simulink model "snell_th"  (R2018b)
settings: Solver=ode8  StartTime=0.0  StopTime=0  RelTol=1e-3
libraries: find6DOFSnell_cl x1
settings Model: Creator=asiddiq2  LastModifiedBy=asiddiq2

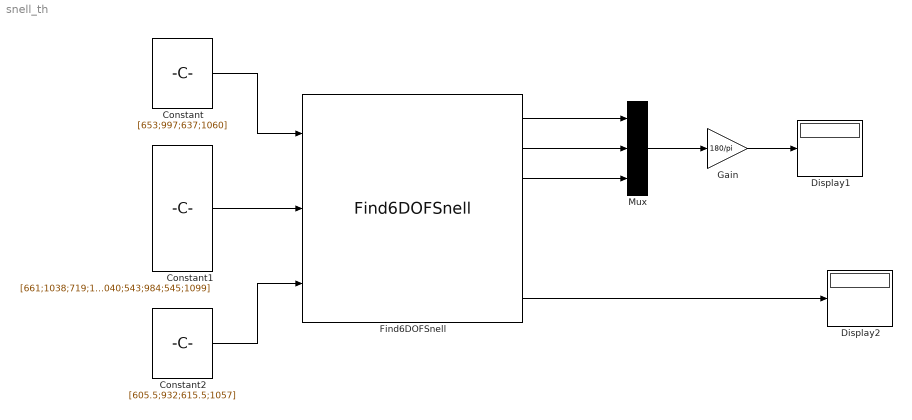
== system snell_th ==
  Constant : Constant  Value=[653;997;637;1060]  VectorParams1D=off
  Constant1 : Constant  Value=[661;1038;719;1040;543;984;545;1099]  VectorParams1D=off
  Constant2 : Constant  Value=[605.5;932;615.5;1057]  VectorParams1D=off
  Display1 : Display
  Display2 : Display
  Find6DOFSnell : find6DOFSnell_cl/Find6DOFSnell  imageDims_px=params.sideImageSize_px.Value  initialCoMPositionVec_cm=params.initCoMPosVec_cm.Value  indxOfRefVec=params.indexOfRefractionAGW.Value  glassThickness_cm=params.glassThickness_cm.Value  prscGlassThick_cm=(3/16)*2.54  cameraFOVAngles_deg=params.cameraFOV_deg.Value  sideEulerAngles_deg=params.sideCamEulAng_deg.Value  sideCamPositionVec_cm=params.sideCamPosVec_cm.Value  sideCamDistToGlass_cm=params.sideDistancetoGlass_cm.Value  botEulerAngles_deg=params.botCamEulAng_deg.Value  botCamPositionVec_cm=params.botCamPosVec_cm.Value  botCamDistToGlass_cm=params.botDistancetoGlass_cm.Value  slantEulerAngles_deg=params.prscpeCamEulAng_deg.Value  slantCamPositionVec_cm=params.prscpeCamPosVec_cm.Value  slantCamDistToGlass_cm=params.prscpeDistancetoGlass_cm.Value  sideSeparation_cm=params.sideDotSepDist_cm.Value  sidePositionVecBF_cm=params.sideDotPosVec_cm.Value  bottomASeparation_cm=params.botADotSepDist_cm.Value  botAPositionVecBF_cm=params.botADotPosVec_cm.Value  bottomBSeparation_cm=params.botBDotSepDist_cm.Value  botBPositionVecBF_cm=params.botBDotPosVec_cm.Value  topSeparation_cm=params.topDotSepDist_cm.Value  topPositionVecBF_cm=params.topDotPosVec_cm.Value
  Gain : Gain  Gain=180/pi
  Mux : Mux  Inputs=3
  wires:
  Constant/1 -> Find6DOFSnell/1
  Constant1/1 -> Find6DOFSnell/2
  Constant2/1 -> Find6DOFSnell/3
  Find6DOFSnell/2 -> Mux/2
  Find6DOFSnell/1 -> Mux/1
  Find6DOFSnell/3 -> Mux/3
  Mux/1 -> Gain/1
  Gain/1 -> Display1/1
  Find6DOFSnell/7 -> Display2/1
